simulink model "sweep_mod3_ciff_3bit"  (Simulink 7.9)
settings: Solver=VariableStepDiscrete  StartTime=0.0  StopTime=simu.trantime  RelTol=1e-3
undefined symbols (not defined in the file): Fs, mod
libraries: dspsigops x3, dspsrcs4 x1
settings Model: Creator=amyles  LastModifiedBy=Arnaldi Isacco
settings DataIOCC: LimitDataPoints=off  MaxDataPoints=50000
settings OptimizationCC: InlineParams=on
settings DebuggingCC: StrictBusMsg=Warning
settings ModelReferenceCC: ModelReferenceNumInstancesAllowed=Single
settings CodeAppCC: CustomSymbolStrType=$N$R$M_T
settings GRTTargetCC: CombineOutputUpdateFcns=off  GRTInterface=on

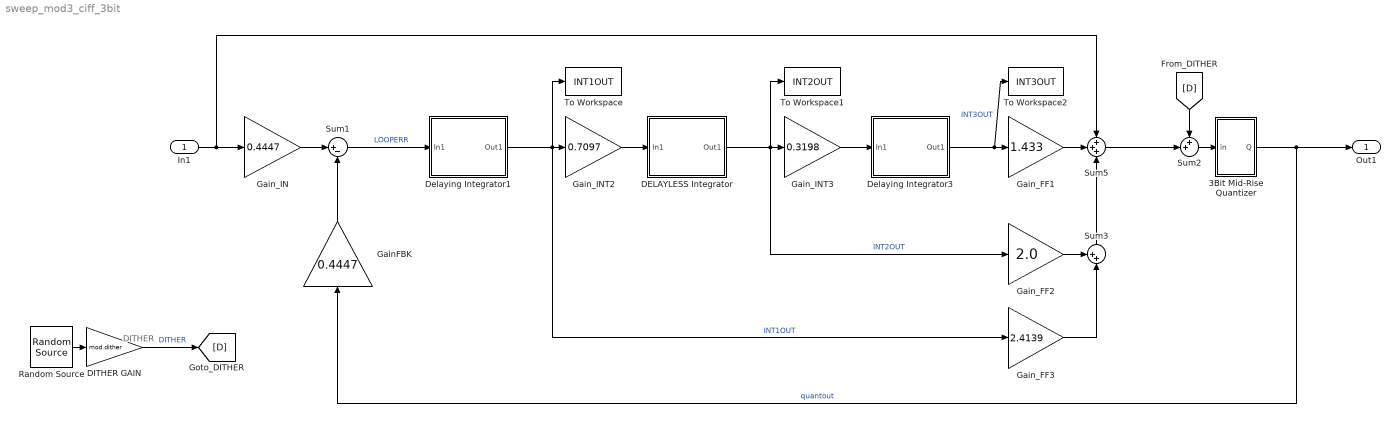
== system sweep_mod3_ciff_3bit ==
  note: DITHER
  In1 : Inport
  3Bit Mid-Rise Quantizer : Subsystem
  DELAYLESS Integrator : Subsystem
  DITHER GAIN : Gain  Gain=mod.dither  SampleTime=1/Fs
  Delaying Integrator1 : Subsystem
  Delaying Integrator3 : Subsystem
  GainFBK : Gain  Gain=0.4447
  Gain_FF1 : Gain  Gain=1.433
  Gain_FF2 : Gain  Gain=2.0
  Gain_FF3 : Gain  Gain=2.4139
  Gain_IN : Gain  Gain=0.4447
  Gain_INT2 : Gain  Gain=0.7097
  Gain_INT3 : Gain  Gain=0.3198
  Random Source : dspsrcs4/Random Source  SrcType=Uniform  NormMethod=Ziggurat  CltLength=12  MinVal=-1  MaxVal=1  MeanVal=0  VarVal=1  RepMode=Not repeatable  rawSeed=1  IsInherit=off  SampMode=Discrete  SampTime=1/Fs  SampFrame=1  DataType=Double  OutComplex=Real
  Sum1 : Sum  Inputs=|+-  SampleTime=1/Fs
      settings: AttributesFormatString=Modulator input\nloop servo error (input - fbk)
  Sum2 : Sum  Inputs=++|
  Sum3 : Sum  Inputs=++|
  Sum5 : Sum  Inputs=+++  SampleTime=1/Fs
  To Workspace : ToWorkspace  VariableName=INT1OUT  SampleTime=-1
  To Workspace1 : ToWorkspace  VariableName=INT2OUT  SampleTime=-1
  To Workspace2 : ToWorkspace  VariableName=INT3OUT  SampleTime=-1
  Out1 : Outport
  wires:
  Sum1/1 -> Delaying Integrator1/1(In1)  "LOOPERR"
  3Bit Mid-Rise Quantizer/1(Q) -> GainFBK/1, Out1/1  "quantout"
  Delaying Integrator1/1(Out1) -> Gain_INT2/1, Gain_FF3/1, To Workspace/1  "INT1OUT"
  Gain_INT2/1 -> DELAYLESS Integrator/1(In1)
  DELAYLESS Integrator/1(Out1) -> Gain_INT3/1, To Workspace1/1, Gain_FF2/1  "INT2OUT"
  GainFBK/1 -> Sum1/2
  Gain_IN/1 -> Sum1/1
  Delaying Integrator3/1(Out1) -> Gain_FF1/1, To Workspace2/1  "INT3OUT"
  Gain_INT3/1 -> Delaying Integrator3/1(In1)
  Gain_FF1/1 -> Sum5/2
  Gain_FF2/1 -> Sum3/1
  Sum3/1 -> Sum5/3
  Gain_FF3/1 -> Sum3/2
  Random Source/1 -> DITHER GAIN/1
  DITHER GAIN/1 -> [D]  "DITHER"
  [D] -> Sum2/1
  Sum2/1 -> 3Bit Mid-Rise Quantizer/1(in)
  Sum5/1 -> Sum2/2
  In1/1 -> Gain_IN/1, Sum5/1

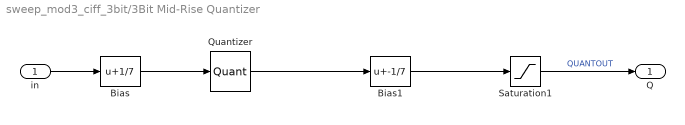
== system sweep_mod3_ciff_3bit/3Bit Mid-Rise Quantizer ==
  in : Inport
  Bias : Bias  Bias=1/7
      settings: AttributesFormatString=Need offset to give\nMID-RISE quantiser
  Bias1 : Bias  Bias=-1/7
  Quantizer : Quantizer  QuantizationInterval=2/7  LinearizeAsGain=off  SampleTime=1/Fs
  Saturation1 : Saturate  UpperLimit=1  LowerLimit=-1
      settings: AttributesFormatString=Limit quantiser\noutput to +/-1
  Q : Outport
  wires:
  Bias/1 -> Quantizer/1
  Quantizer/1 -> Bias1/1
  Bias1/1 -> Saturation1/1
  in/1 -> Bias/1
  Saturation1/1 -> Q/1  "QUANTOUT"

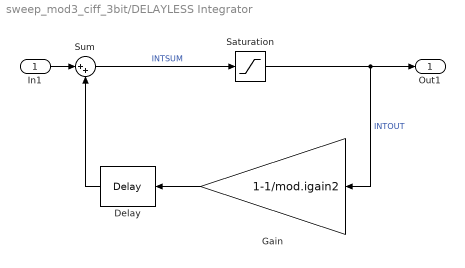
== system sweep_mod3_ciff_3bit/DELAYLESS Integrator ==
  In1 : Inport
  Delay : dspsigops/Delay  InputProcessing=Inherited (this choice will be removed - see release notes)  dly_unit=Samples  delay=1  ic_detail=off  dif_ic_for_ch=off  dif_ic_for_dly=off  ic=0  reset_popup=None
  Gain : Gain  Gain=1-1/mod.igain2
      settings: AttributesFormatString=Integrator leakage
  Saturation : Saturate  UpperLimit=mod.isat2  LowerLimit=-(mod.isat2)
  Sum : Sum  Inputs=|++
      settings: AttributesFormatString=Integrator summer
  Out1 : Outport
  wires:
  In1/1 -> Sum/1
  Saturation/1 -> Out1/1, Gain/1  "INTOUT"
  Gain/1 -> Delay/1
  Sum/1 -> Saturation/1  "INTSUM"
  Delay/1 -> Sum/2

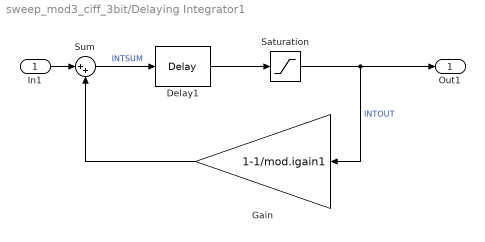
== system sweep_mod3_ciff_3bit/Delaying Integrator1 ==
  In1 : Inport
  Delay1 : dspsigops/Delay  InputProcessing=Inherited (this choice will be removed - see release notes)  dly_unit=Samples  delay=1  ic_detail=off  dif_ic_for_ch=off  dif_ic_for_dly=off  ic=0  reset_popup=None
  Gain : Gain  Gain=1-1/mod.igain1
      settings: AttributesFormatString=Integrator leakage
  Saturation : Saturate  UpperLimit=mod.isat1  LowerLimit=-(mod.isat1)
  Sum : Sum  Inputs=|++
      settings: AttributesFormatString=Integrator summer
  Out1 : Outport
  wires:
  Sum/1 -> Delay1/1  "INTSUM"
  Gain/1 -> Sum/2
  Saturation/1 -> Gain/1, Out1/1  "INTOUT"
  In1/1 -> Sum/1
  Delay1/1 -> Saturation/1

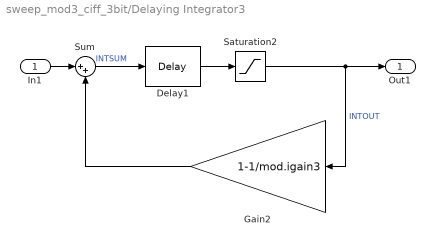
== system sweep_mod3_ciff_3bit/Delaying Integrator3 ==
  In1 : Inport
  Delay1 : dspsigops/Delay  InputProcessing=Inherited (this choice will be removed - see release notes)  dly_unit=Samples  delay=1  ic_detail=off  dif_ic_for_ch=off  dif_ic_for_dly=off  ic=0  reset_popup=None
  Gain2 : Gain  Gain=1-1/mod.igain3
      settings: AttributesFormatString=Integrator leakage
  Saturation2 : Saturate  UpperLimit=mod.isat3  LowerLimit=-(mod.isat3)
  Sum : Sum  Inputs=|++
      settings: AttributesFormatString=Integrator summer
  Out1 : Outport
  wires:
  Sum/1 -> Delay1/1  "INTSUM"
  Gain2/1 -> Sum/2
  Saturation2/1 -> Gain2/1, Out1/1  "INTOUT"
  In1/1 -> Sum/1
  Delay1/1 -> Saturation2/1
